simulink model "H8_6GDL_nolineal_desactualizado"  (R2022b)
settings: Solver=VariableStepAuto  StartTime=0.0  StopTime=3  MaxStep=1e-3  RelTol=1e-3
InitFcn:
  | %load("ems.mat");
  | %load("hems.mat");
  | %load("Ka.mat");
  | load('fuerzasY_LIM.mat')
  | load('matrices_linealizacion_6gdl.mat')
  | m = 200;
  | g = 9.81;
  | 
  | x_lev12 = 0.443;
  | x_lev34 = 0.542;%0.443;
  | x_guid12 = 0.4475;
  | x_guid34 = 0.5465;
  | x_lim = 0.0495;
  | 
  | y_lev13 = 0.23686;
  | y_lev24 = 0.23686;
  | y_guid13 = 0.24263;
  | y_guid24 = 0.24263;
  | y_lim = 0.0005;
  | y_brk = 0.21552;
  | 
  | z_lev = 0.08546;
  | z_guid = 0.026;
  | z_lim = 0.1055;
  | z_brk = 0.03941;
  | 
  | kp_lev = 50;
  | ki_lev = 400;
  | kp_guid = 6;
  | ki_guid = 46.5;
  | 
  | Imax_lev = 50;
  | Imin_lev = -50;
  | Imax_guid = 50;
  | Imin_guid = 0;
  | 
  | cg_nom=0.567;
  | lev_nom=0.01965;
  | cg_suelo=0.56985;
  | cg_techo=0.55735;
  | 
  | I = [43.082 0 0; 0 26.887 -0; 0 0 29.297]
values from neighbouring files (symbols this model uses):
  A6 = [0 0 0 0 0 0 0 0 0 0 0 0 ... (100 elements, 10x10)]    [matrices_linealizacion_6gdl.mat]
  B6 = [0 0 0 0 0 0.000575563603666 -0.0459993641186 -0.0505103975277 0.151580453785 0.00175830093621 0 0 ... (80 elements, 10x8)]    [matrices_linealizacion_6gdl.mat]
  C6 = [1 0 0 0 0 0 0 0 0 0 0 1 ... (100 elements, 10x10)]    [matrices_linealizacion_6gdl.mat]
  current = [0 10 20 30 40 50 60 70 80 90 100]    [fuerzasY_LIM.mat]
  D6 = [0 0 0 0 0 0 0 0 0 0 0 0 ... (80 elements, 10x8)]    [matrices_linealizacion_6gdl.mat]
  Ka = [34.5916764023 4.46928641015 34.7816336405 4.65924364837 92.2484067139 -92.2484067139 74.2332308826 -74.2332308826 -4220.94514487 -4209.6309051 -4205.06787146 -4193.7536317 ... (120 elements, 8x15)]    [Ka.mat]    (also in linealizacion_5gdl_bien.m = place(Aa,Ba,[ -1.5 -1.5 -1.5 -1.5 -2 -2 -6 -6 -7 -7 -5 -5 -2; linealizacion_EMS.m = place(Aa,Ba,[ -1 -1 -2 -2 -3 -3 -6 -6 -7 -7 -5 -5 -4 -4 -5 -)
  Y = [0 1 2 3 4 5 6]    [fuerzasY_LIM.mat]
undefined symbols (not defined in the file or in its folder): ems, FuerzaRail_Y, hems, magnitude
libraries: slpidlib x16
(part 2 of 2)

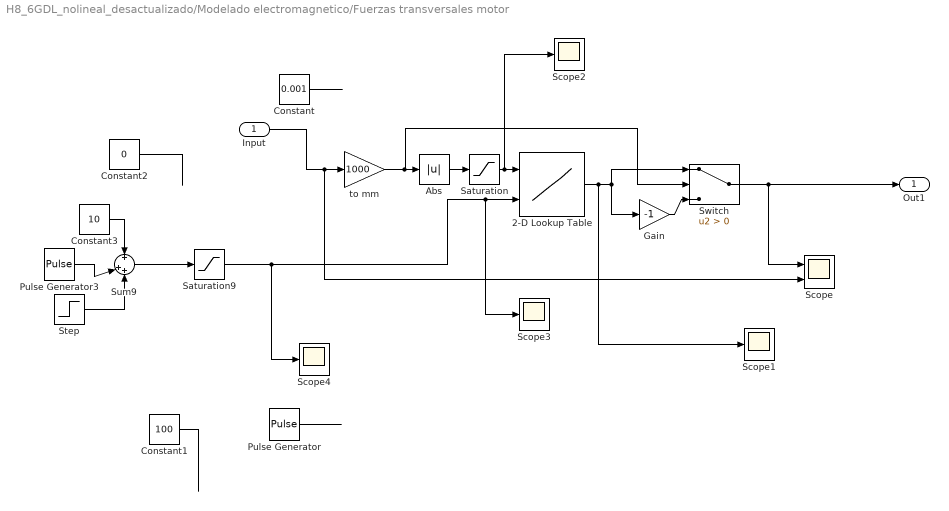
== system H8_6GDL_nolineal_desactualizado/Modelado electromagnetico/Fuerzas transversales motor ==
  Input : Inport
  2-D Lookup Table : Lookup_n-D  BreakpointsForDimension1=Y  BreakpointsForDimension2=current  Table=FuerzaRail_Y  InternalRulePriority=Speed  RndMeth=Simplest
      settings: InputPortMap=u0,u1
  Abs : Abs  SaturateOnIntegerOverflow=off
  Constant : Constant  Value=0.001
  Constant1 : Constant  Value=100
  Constant2 : Constant  Value=0
  Constant3 : Constant  Value=10
  Gain : Gain  Gain=-1
  Pulse Generator : DiscretePulseGenerator  PulseType=Time based  Amplitude=100  PulseWidth=75  PhaseDelay=3
  Pulse Generator3 : DiscretePulseGenerator  PulseType=Time based  Amplitude=100  PulseWidth=95  PhaseDelay=4.2
  Saturation : Saturate  UpperLimit=6  LowerLimit=0
  Saturation9 : Saturate  UpperLimit=100  LowerLimit=0
  Scope : Scope  NumInputPorts=2
  Scope{1..4} (4 alike) : Scope
  Step : Step  Time=8.2  After=-100  SampleTime=0
  Sum9 : Sum  Inputs=+|++
  Switch : Switch  Criteria=u2 > Threshold  SaturateOnIntegerOverflow=off  InputSameDT=off
  to mm : Gain  Gain=1000
  Out1 : Outport
  wires:
  Constant/1 -> ?
  Input/1 -> to mm/1, Scope/2
  Gain/1 -> Switch/3
  Abs/1 -> Saturation/1
  to mm/1 -> Switch/2, Abs/1
  2-D Lookup Table/1 -> Scope1/1, Gain/1, Switch/1
  Saturation9/1 -> Scope4/1, Scope3/1, 2-D Lookup Table/2
  Switch/1 -> Out1/1, Scope/1
  Saturation/1 -> Scope2/1, 2-D Lookup Table/1
  Pulse Generator/1 -> ?
  Constant1/1 -> ?
  Constant2/1 -> ?
  Sum9/1 -> Saturation9/1
  Pulse Generator3/1 -> Sum9/2
  Constant3/1 -> Sum9/1
  Step/1 -> Sum9/3

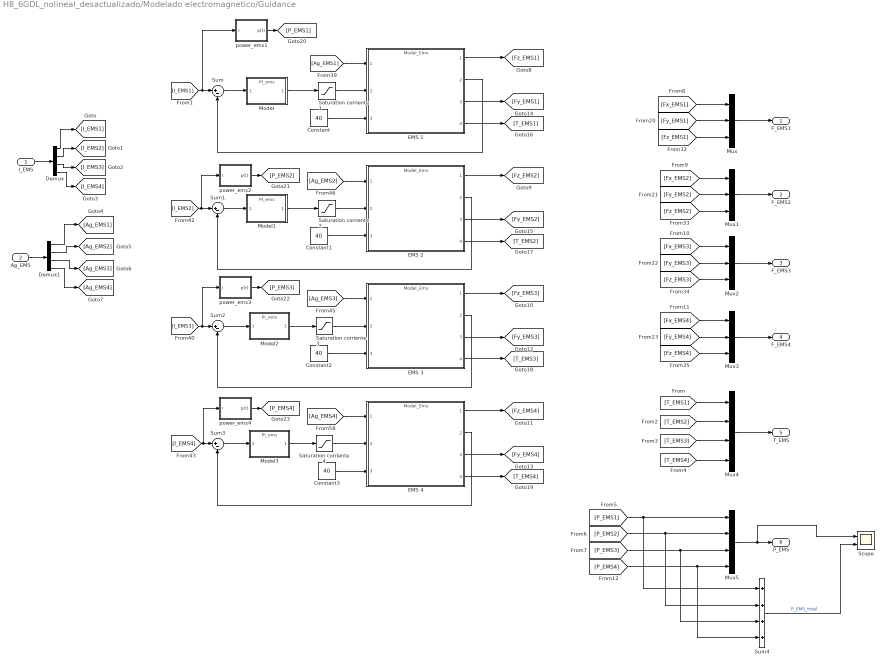
== system H8_6GDL_nolineal_desactualizado/Modelado electromagnetico/Guidance ==
  I_EMS : Inport
  Ag_EMS : Inport  Port=2
  Constant{,1..3} (4 alike) : Constant  Value=40
  Demux : Demux
  Demux1 : Demux
  EMS {1..4} (4 alike) : ModelReference  ModelNameDialog=Model_Ems.slx  SimulationMode=Normal  ModelReferenceVersion=1.21
  Model{,1..3} (4 alike) : ModelReference  ModelNameDialog=PI_ems.slx  SimulationMode=Normal  ModelReferenceVersion=1.2
  Mux{,1..3} (4 alike) : Mux  Inputs=3
  Mux4 : Mux
  Mux5 : Mux
  Saturation corriente {1..4} (4 alike) : Saturate  UpperLimit=Imax_guid  LowerLimit=Imin_guid
  Scope : Scope  NumInputPorts=2
  Sum{,1..3} (4 alike) : Sum  Inputs=|+-
  Sum4 : Sum  Inputs=++++
  power_ems1 : Subsystem
  power_ems2 : Subsystem
  power_ems3 : Subsystem
  power_ems4 : Subsystem
  F_EMS1 : Outport
  F_EMS2 : Outport  Port=2
  F_EMS3 : Outport  Port=3
  F_EMS4 : Outport  Port=4
  T_EMS : Outport  Port=5
  P_EMS : Outport  Port=6
  wires:
  [Fz_EMS4] -> Mux3/3
  Demux1/4 -> [Ag_EMS4]
  [Fy_EMS1] -> Mux/2
  I_EMS/1 -> Demux/1
  Mux1/1 -> F_EMS2/1
  Demux/2 -> [I_EMS2]
  [Fy_EMS3] -> Mux2/2
  Mux3/1 -> F_EMS4/1
  [Fy_EMS4] -> Mux3/2
  [Fz_EMS1] -> Mux/3
  Mux/1 -> F_EMS1/1
  Mux2/1 -> F_EMS3/1
  [Fx_EMS3] -> Mux2/1
  Demux1/3 -> [Ag_EMS3]
  Ag_EMS/1 -> Demux1/1
  [Fz_EMS3] -> Mux2/3
  Demux/1 -> [I_EMS1]
  [Fz_EMS2] -> Mux1/3
  [Fx_EMS1] -> Mux/1
  Demux1/1 -> [Ag_EMS1]
  Demux/4 -> [I_EMS4]
  [Fx_EMS2] -> Mux1/1
  [Fy_EMS2] -> Mux1/2
  [Fx_EMS4] -> Mux3/1
  Demux/3 -> [I_EMS3]
  Demux1/2 -> [Ag_EMS2]
  EMS 1/3 -> [Fy_EMS1]
  [Ag_EMS4] -> EMS 4/1
  EMS 4/3 -> [Fy_EMS4]
  EMS 4/1 -> [Fz_EMS4]
  EMS 2/1 -> [Fz_EMS2]
  EMS 1/2 -> Sum/2
  EMS 3/1 -> [Fz_EMS3]
  [Ag_EMS3] -> EMS 3/1
  Constant1/1 -> EMS 2/3
  Constant3/1 -> EMS 4/3
  Constant2/1 -> EMS 3/3
  Constant/1 -> EMS 1/3
  EMS 1/1 -> [Fz_EMS1]
  [Ag_EMS2] -> EMS 2/1
  Model/1 -> Saturation corriente 1/1
  EMS 3/3 -> [Fy_EMS3]
  EMS 2/3 -> [Fy_EMS2]
  [Ag_EMS1] -> EMS 1/1
  Sum/1 -> Model/1
  Sum1/1 -> Model1/1
  EMS 2/2 -> Sum1/2
  [I_EMS2] -> power_ems2/1(I), Sum1/1
  Model1/1 -> Saturation corriente 2/1
  [I_EMS1] -> power_ems1/1(I), Sum/1
  Sum2/1 -> Model2/1
  EMS 3/2 -> Sum2/2
  [I_EMS3] -> power_ems3/1(I), Sum2/1
  Model2/1 -> Saturation corriente 3/1
  Sum3/1 -> Model3/1
  EMS 4/2 -> Sum3/2
  [I_EMS4] -> power_ems4/1(I), Sum3/1
  Model3/1 -> Saturation corriente 4/1
  Mux4/1 -> T_EMS/1
  EMS 1/4 -> [T_EMS1]
  EMS 2/4 -> [T_EMS2]
  EMS 3/4 -> [T_EMS3]
  EMS 4/4 -> [T_EMS4]
  [T_EMS1] -> Mux4/1
  [T_EMS2] -> Mux4/2
  [T_EMS3] -> Mux4/3
  [T_EMS4] -> Mux4/4
  Saturation corriente 1/1 -> EMS 1/2
  Saturation corriente 2/1 -> EMS 2/2
  Saturation corriente 3/1 -> EMS 3/2
  Saturation corriente 4/1 -> EMS 4/2
  power_ems1/1(p(t)) -> [P_EMS1]
  power_ems2/1(p(t)) -> [P_EMS2]
  power_ems3/1(p(t)) -> [P_EMS3]
  power_ems4/1(p(t)) -> [P_EMS4]
  [P_EMS4] -> Sum4/4, Mux5/4
  [P_EMS1] -> Mux5/1, Sum4/1
  Sum4/1 -> Scope/2  "P_EMS_total"
  [P_EMS2] -> Mux5/2, Sum4/2
  Mux5/1 -> Scope/1, P_EMS/1
  [P_EMS3] -> Sum4/3, Mux5/3

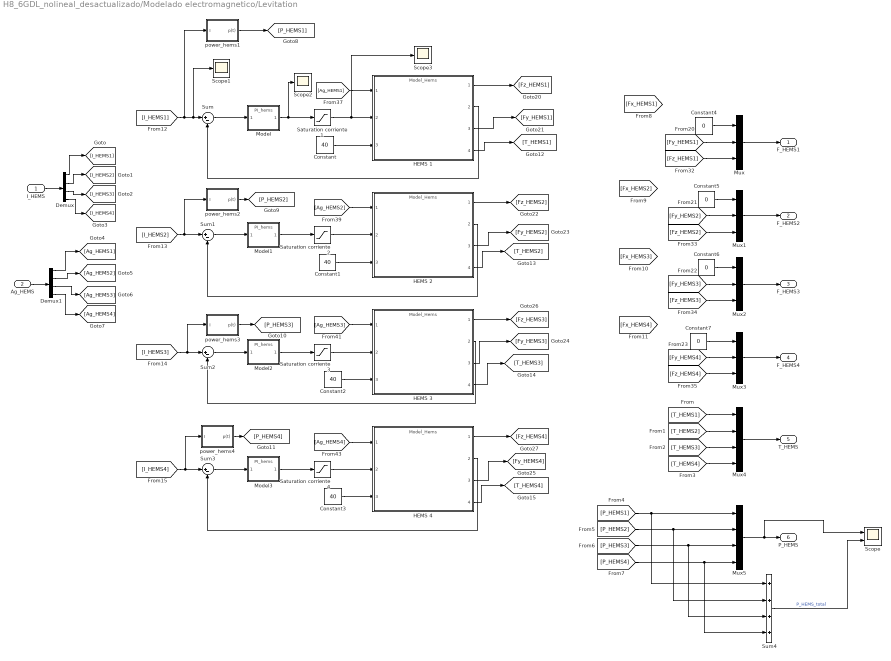
== system H8_6GDL_nolineal_desactualizado/Modelado electromagnetico/Levitation ==
  I_HEMS : Inport
  Ag_HEMS : Inport  Port=2
  Constant{,1..3} (4 alike) : Constant  Value=40
  Constant{4..7} (4 alike) : Constant  Value=0
  Demux : Demux
  Demux1 : Demux
  HEMS {1..4} (4 alike) : ModelReference  ModelNameDialog=Model_Hems.slx  SimulationMode=Normal  ModelReferenceVersion=1.19
  Model{,1..3} (4 alike) : ModelReference  ModelNameDialog=PI_hems.slx  SimulationMode=Normal  ModelReferenceVersion=1.3
  Mux{,1..3} (4 alike) : Mux  Inputs=3
  Mux4 : Mux
  Mux5 : Mux
  Saturation corriente {1..4} (4 alike) : Saturate  UpperLimit=Imax_lev  LowerLimit=Imin_lev
  Scope : Scope  NumInputPorts=2
  Scope1 : Scope
  Scope2 : Scope
  Scope3 : Scope
  Sum{,1..3} (4 alike) : Sum  Inputs=|+-
  Sum4 : Sum  Inputs=++++
  power_hems1 : Subsystem
  power_hems2 : Subsystem
  power_hems3 : Subsystem
  power_hems4 : Subsystem
  F_HEMS1 : Outport
  F_HEMS2 : Outport  Port=2
  F_HEMS3 : Outport  Port=3
  F_HEMS4 : Outport  Port=4
  T_HEMS : Outport  Port=5
  P_HEMS : Outport  Port=6
  wires:
  I_HEMS/1 -> Demux/1
  Mux/1 -> F_HEMS1/1
  Mux1/1 -> F_HEMS2/1
  Mux2/1 -> F_HEMS3/1
  Mux3/1 -> F_HEMS4/1
  Demux/1 -> [I_HEMS1]
  Demux/2 -> [I_HEMS2]
  Demux/3 -> [I_HEMS3]
  Demux/4 -> [I_HEMS4]
  Demux1/2 -> [Ag_HEMS2]
  Demux1/3 -> [Ag_HEMS3]
  Ag_HEMS/1 -> Demux1/1
  Demux1/4 -> [Ag_HEMS4]
  Demux1/1 -> [Ag_HEMS1]
  Constant4/1 -> Mux/1
  Constant5/1 -> Mux1/1
  Constant6/1 -> Mux2/1
  Constant7/1 -> Mux3/1
  [Fy_HEMS1] -> Mux/2
  [Fy_HEMS2] -> Mux1/2
  [Fy_HEMS3] -> Mux2/2
  [Fy_HEMS4] -> Mux3/2
  [Fz_HEMS1] -> Mux/3
  [Fz_HEMS2] -> Mux1/3
  [Fz_HEMS3] -> Mux2/3
  [Fz_HEMS4] -> Mux3/3
  Model/1 -> Scope2/1, Saturation corriente 1/1
  [Ag_HEMS1] -> HEMS 1/1
  HEMS 1/1 -> [Fz_HEMS1]
  HEMS 1/3 -> [Fy_HEMS1]
  HEMS 2/3 -> [Fy_HEMS2]
  HEMS 2/1 -> [Fz_HEMS2]
  [Ag_HEMS2] -> HEMS 2/1
  Model1/1 -> Saturation corriente 2/1
  HEMS 3/3 -> [Fy_HEMS3]
  HEMS 3/1 -> [Fz_HEMS3]
  [Ag_HEMS3] -> HEMS 3/1
  Model2/1 -> Saturation corriente 3/1
  HEMS 4/3 -> [Fy_HEMS4]
  HEMS 4/1 -> [Fz_HEMS4]
  [Ag_HEMS4] -> HEMS 4/1
  Model3/1 -> Saturation corriente 4/1
  Constant1/1 -> HEMS 2/3
  Constant2/1 -> HEMS 3/3
  Constant3/1 -> HEMS 4/3
  HEMS 1/2 -> Sum/2
  Sum/1 -> Model/1
  Sum1/1 -> Model1/1
  HEMS 2/2 -> Sum1/2
  Sum2/1 -> Model2/1
  HEMS 3/2 -> Sum2/2
  Sum3/1 -> Model3/1
  HEMS 4/2 -> Sum3/2
  [I_HEMS1] -> power_hems1/1(I), Scope1/1, Sum/1
  [I_HEMS2] -> power_hems2/1(I), Sum1/1
  [I_HEMS3] -> power_hems3/1(I), Sum2/1
  [I_HEMS4] -> power_hems4/1(I), Sum3/1
  HEMS 1/4 -> [T_HEMS1]
  Constant/1 -> HEMS 1/3
  HEMS 2/4 -> [T_HEMS2]
  HEMS 3/4 -> [T_HEMS3]
  HEMS 4/4 -> [T_HEMS4]
  Mux4/1 -> T_HEMS/1
  [T_HEMS1] -> Mux4/1
  [T_HEMS4] -> Mux4/4
  [T_HEMS3] -> Mux4/3
  [T_HEMS2] -> Mux4/2
  Saturation corriente 1/1 -> Scope3/1, HEMS 1/2
  Saturation corriente 2/1 -> HEMS 2/2
  Saturation corriente 3/1 -> HEMS 3/2
  Saturation corriente 4/1 -> HEMS 4/2
  power_hems1/1(p(t)) -> [P_HEMS1]
  [P_HEMS4] -> Sum4/4, Mux5/4
  [P_HEMS2] -> Mux5/2, Sum4/2
  [P_HEMS3] -> Sum4/3, Mux5/3
  Mux5/1 -> Scope/1, P_HEMS/1
  [P_HEMS1] -> Mux5/1, Sum4/1
  Sum4/1 -> Scope/2  "P_HEMS_total"
  power_hems2/1(p(t)) -> [P_HEMS2]
  power_hems3/1(p(t)) -> [P_HEMS3]
  power_hems4/1(p(t)) -> [P_HEMS4]

== system H8_6GDL_nolineal_desactualizado/Control/state space control/Moving Average Filter ==
  input : Inport
  Delay : Delay  DelayLength=M  SampleTime=fs
  Delay1 : Delay  DelayLength=1  SampleTime=fs
  Gain : Gain  Gain=1/M
  Sum : Sum  Inputs=|+-
  Sum1 : Sum  Inputs=|++
  output : Outport
  wires:
  input/1 -> Delay/1, Sum/1
  Delay/1 -> Sum/2
  Sum/1 -> Sum1/1
  Sum1/1 -> Delay1/1, Gain/1
  Delay1/1 -> Sum1/2
  Gain/1 -> output/1

== system H8_6GDL_nolineal_desactualizado/Control/state space control/Moving Average Filter1 ==
  input : Inport
  Delay : Delay  DelayLength=M  SampleTime=fs
  Delay1 : Delay  DelayLength=1  SampleTime=fs
  Gain : Gain  Gain=1/M
  Sum : Sum  Inputs=|+-
  Sum1 : Sum  Inputs=|++
  output : Outport
  wires:
  input/1 -> Delay/1, Sum/1
  Delay/1 -> Sum/2
  Sum/1 -> Sum1/1
  Sum1/1 -> Delay1/1, Gain/1
  Delay1/1 -> Sum1/2
  Gain/1 -> output/1

== system H8_6GDL_nolineal_desactualizado/Control/state space control/Moving Average Filter2 ==
  input : Inport
  Delay : Delay  DelayLength=M  SampleTime=fs
  Delay1 : Delay  DelayLength=1  SampleTime=fs
  Gain : Gain  Gain=1/M
  Sum : Sum  Inputs=|+-
  Sum1 : Sum  Inputs=|++
  output : Outport
  wires:
  input/1 -> Delay/1, Sum/1
  Delay/1 -> Sum/2
  Sum/1 -> Sum1/1
  Sum1/1 -> Delay1/1, Gain/1
  Delay1/1 -> Sum1/2
  Gain/1 -> output/1

== system H8_6GDL_nolineal_desactualizado/Control/state space control/Moving Average Filter3 ==
  input : Inport
  Delay : Delay  DelayLength=M  SampleTime=fs
  Delay1 : Delay  DelayLength=1  SampleTime=fs
  Gain : Gain  Gain=1/M
  Sum : Sum  Inputs=|+-
  Sum1 : Sum  Inputs=|++
  output : Outport
  wires:
  input/1 -> Delay/1, Sum/1
  Delay/1 -> Sum/2
  Sum/1 -> Sum1/1
  Sum1/1 -> Delay1/1, Gain/1
  Delay1/1 -> Sum1/2
  Gain/1 -> output/1

== system H8_6GDL_nolineal_desactualizado/Control/state space control/Moving Average Filter4 ==
  input : Inport
  Delay : Delay  DelayLength=M  SampleTime=fs
  Delay1 : Delay  DelayLength=1  SampleTime=fs
  Gain : Gain  Gain=1/M
  Sum : Sum  Inputs=|+-
  Sum1 : Sum  Inputs=|++
  output : Outport
  wires:
  input/1 -> Delay/1, Sum/1
  Delay/1 -> Sum/2
  Sum/1 -> Sum1/1
  Sum1/1 -> Delay1/1, Gain/1
  Delay1/1 -> Sum1/2
  Gain/1 -> output/1

== system H8_6GDL_nolineal_desactualizado/EMS/RL/Subsystem ==
  Current : Inport
  Temperature : Inport  Port=2
  Resistance : Constant  Value=ems.Resistance
  R : Outport
  wires:
  Resistance/1 -> R/1

== system H8_6GDL_nolineal_desactualizado/EMS/RL1/Subsystem ==
  Current : Inport
  Temperature : Inport  Port=2
  Resistance : Constant  Value=ems.Resistance
  R : Outport
  wires:
  Resistance/1 -> R/1

== system H8_6GDL_nolineal_desactualizado/EMS/RL2/Subsystem ==
  Current : Inport
  Temperature : Inport  Port=2
  Resistance : Constant  Value=ems.Resistance
  R : Outport
  wires:
  Resistance/1 -> R/1

== system H8_6GDL_nolineal_desactualizado/EMS/RL3/Subsystem ==
  Current : Inport
  Temperature : Inport  Port=2
  Resistance : Constant  Value=ems.Resistance
  R : Outport
  wires:
  Resistance/1 -> R/1

== system H8_6GDL_nolineal_desactualizado/HEMS/RL/Subsystem ==
  Current : Inport
  Temperature : Inport  Port=2
  Resistance : Constant  Value=hems.Resistance
  R : Outport
  wires:
  Resistance/1 -> R/1

== system H8_6GDL_nolineal_desactualizado/HEMS/RL1/Subsystem ==
  Current : Inport
  Temperature : Inport  Port=2
  Resistance : Constant  Value=hems.Resistance
  R : Outport
  wires:
  Resistance/1 -> R/1

== system H8_6GDL_nolineal_desactualizado/HEMS/RL2/Subsystem ==
  Current : Inport
  Temperature : Inport  Port=2
  Resistance : Constant  Value=hems.Resistance
  R : Outport
  wires:
  Resistance/1 -> R/1

== system H8_6GDL_nolineal_desactualizado/HEMS/RL3/Subsystem ==
  Current : Inport
  Temperature : Inport  Port=2
  Resistance : Constant  Value=hems.Resistance
  R : Outport
  wires:
  Resistance/1 -> R/1

== system H8_6GDL_nolineal_desactualizado/Modelado electromagnetico/Guidance/power_ems1 ==
  I : Inport
  Constant8 : Constant  Value=ems.Resistance
  Power : Math  Operator=magnitude^2
  Product : Product
  p(t) : Outport
  wires:
  I/1 -> Power/1
  Product/1 -> p(t)/1
  Power/1 -> Product/1
  Constant8/1 -> Product/2

== system H8_6GDL_nolineal_desactualizado/Modelado electromagnetico/Guidance/power_ems2 ==
  I : Inport
  Constant8 : Constant  Value=ems.Resistance
  Power : Math  Operator=magnitude^2
  Product : Product
  p(t) : Outport
  wires:
  I/1 -> Power/1
  Product/1 -> p(t)/1
  Power/1 -> Product/1
  Constant8/1 -> Product/2

== system H8_6GDL_nolineal_desactualizado/Modelado electromagnetico/Guidance/power_ems3 ==
  I : Inport
  Constant8 : Constant  Value=ems.Resistance
  Power : Math  Operator=magnitude^2
  Product : Product
  p(t) : Outport
  wires:
  I/1 -> Power/1
  Product/1 -> p(t)/1
  Power/1 -> Product/1
  Constant8/1 -> Product/2

== system H8_6GDL_nolineal_desactualizado/Modelado electromagnetico/Guidance/power_ems4 ==
  I : Inport
  Constant8 : Constant  Value=ems.Resistance
  Power : Math  Operator=magnitude^2
  Product : Product
  p(t) : Outport
  wires:
  I/1 -> Power/1
  Product/1 -> p(t)/1
  Power/1 -> Product/1
  Constant8/1 -> Product/2

== system H8_6GDL_nolineal_desactualizado/Modelado electromagnetico/Levitation/power_hems1 ==
  I : Inport
  Constant8 : Constant  Value=hems.Resistance
  Power : Math  Operator=magnitude^2
  Product : Product
  p(t) : Outport
  wires:
  I/1 -> Power/1
  Product/1 -> p(t)/1
  Power/1 -> Product/1
  Constant8/1 -> Product/2

== system H8_6GDL_nolineal_desactualizado/Modelado electromagnetico/Levitation/power_hems2 ==
  I : Inport
  Constant8 : Constant  Value=hems.Resistance
  Power : Math  Operator=magnitude^2
  Product : Product
  p(t) : Outport
  wires:
  I/1 -> Power/1
  Product/1 -> p(t)/1
  Power/1 -> Product/1
  Constant8/1 -> Product/2

== system H8_6GDL_nolineal_desactualizado/Modelado electromagnetico/Levitation/power_hems3 ==
  I : Inport
  Constant8 : Constant  Value=hems.Resistance
  Power : Math  Operator=magnitude^2
  Product : Product
  p(t) : Outport
  wires:
  I/1 -> Power/1
  Product/1 -> p(t)/1
  Power/1 -> Product/1
  Constant8/1 -> Product/2

== system H8_6GDL_nolineal_desactualizado/Modelado electromagnetico/Levitation/power_hems4 ==
  I : Inport
  Constant8 : Constant  Value=hems.Resistance
  Power : Math  Operator=magnitude^2
  Product : Product
  p(t) : Outport
  wires:
  I/1 -> Power/1
  Product/1 -> p(t)/1
  Power/1 -> Product/1
  Constant8/1 -> Product/2
